simulink model "Conv_GripIntrlck"  (R2016b)
settings: configuration reference "CodeGenConfigSet" (kept outside this file)
libraries: simulink x1
settings Model: Creator=Wollf  LastModifiedBy=Wollf
settings ConfigSetRef: SourceLocation=Base Workspace

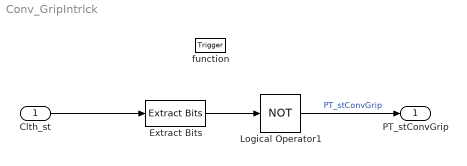
== system Conv_GripIntrlck ==
  Clth_st : Inport  Description=Clutch information  OutMin=0  OutMax=255  OutDataTypeStr=State_uint8
  function : TriggerPort  TriggerType=function-call  VariantControl=Variant
  Extract Bits : simulink/Logic and Bit Operations/Extract Bits  bitsToExtract=Range of bits  numBits=8  bitIdxRange=0  outScalingMode=Treat bit field as an integer
  Logical Operator1 : Logic  Operator=NOT  AllPortsSameDT=off  OutDataTypeStr=boolean
  PT_stConvGrip : Outport  Description=Grip status clutch  OutMin=0  OutMax=1  OutDataTypeStr=boolean
  wires:
  Logical Operator1/1 -> PT_stConvGrip/1  "PT_stConvGrip"
  Extract Bits/1 -> Logical Operator1/1
  Clth_st/1 -> Extract Bits/1
